simulink model "testLoadDataFromFiles"  (R2021b)
settings: Solver=VariableStepAuto  StartTime=0.0  StopTime=inf  RelTol=1e-3
model workspace (MATLAB code in the model file):
  | % Test using the TCT auto-generated files.
  | utils = StateMachineUtils;
  | 
  | utils = utils.loadEventsInAds('resources/tct/ALLEVENT.ADS');
  | 
  | utils = utils.loadDisabledEventsInPdt('resources/tct/DATA_SIMSUP1_MG1.PDT');
  | 
  | utils = utils.loadTransitionsInAds('resources/tct/SIMSUP1_MG1.ADS');
  | 
  | stateMatrix = StateEncoder.encode(utils.statesArray);
  | 
  | transitions = utils.transitions;
  | 
  | eventsArray = utils.eventsArray;
libraries: simulink x1
settings Model: Creator=andrerangel  LastModifiedBy=andrerangel

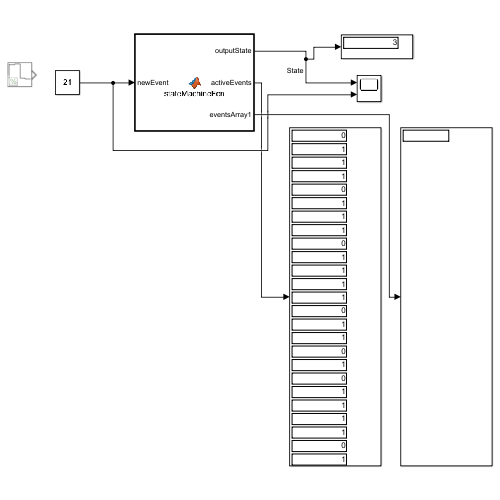
[thumbnail: Simulink's stored preview of the top-level diagram]
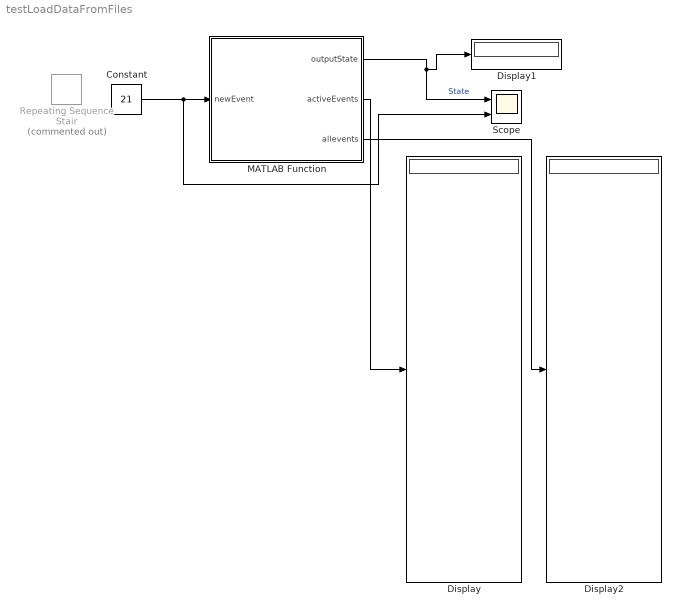
== system testLoadDataFromFiles ==
  Constant : Constant  Value=21
  Display : Display
  Display1 : Display
  Display2 : Display
  MATLAB Function : MATLAB Function  TreatAsAtomicUnit=on
  Repeating Sequence Stair : simulink/Sources/Repeating Sequence Stair  Commented=on  OutValues="[31 32  12 11]"  tsamp=-1  OutMin=[]  OutMax=[]  OutDataTypeStr=double  OutputDataTypeScalingMode=double  OutDataType=fixdt(0,8)  ConRadixGroup=Best Precision: Vector-wise  OutScaling=2^-12
  Scope : Scope  NumInputPorts=2
  wires:
  MATLAB Function/1(outputState) -> Display1/1, Scope/1  "State"
  MATLAB Function/2(activeEvents) -> Display/1
  Constant/1 -> Scope/2, MATLAB Function/1(newEvent)
  MATLAB Function/3(allevents) -> Display2/1

== matlab function testLoadDataFromFiles/MATLAB Function ==
  data: newEvent input; outputState output size=[1 1]; stateMatrix parameter; transitions parameter; eventsArray parameter; activeEvents output; allevents output
function [outputState, activeEvents, allevents] = stateMachineFcn(newEvent, stateMatrix, transitions, eventsArray)
% Test of a State Machine with data from files.

% Initialize a persistent object. Its value will not be erased as this
% block finishes.
persistent stateMachine

% Assign the persistent object to the StateMachine class with data passed
% as parameters.
if (isempty(stateMachine))
    statesArray = StateEncoder.decode(stateMatrix);
    stateMachine = StateMachine(statesArray, transitions, eventsArray);
end

stateMachine.inputEvent = newEvent;
outputState = stateMachine.currentState.number;
activeEvents = stateMachine.currentState.activeEvents;
allevents = stateMachine.eventsArray;
